simulink model "hw6"  (R2017a)
settings: Solver=VariableStepAuto  StartTime=0.0  StopTime=10.0  RelTol=1e-3
settings Model: Creator=Jessica  LastModifiedBy=Jessica

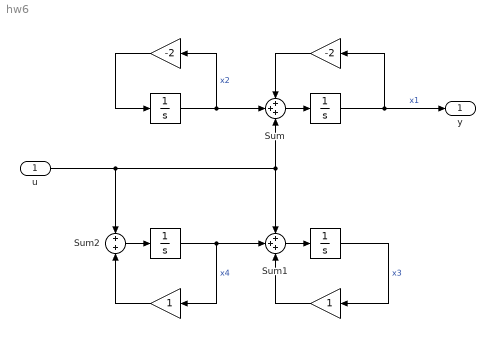
== system hw6 ==
  u : Inport
  " " : Gain  Gain=-2
  "  " : Integrator
  "   " : Integrator
  "    " : Gain  Gain=-2
  "      " : Integrator
  "       " : Gain
  "        " : Gain
  "         " : Integrator
  Sum : Sum  Inputs=+++
  Sum1 : Sum  Inputs=+++
  Sum2 : Sum  Inputs=+|+
  y : Outport
  wires:
  "        "/1 -> Sum2/2
  "         "/1 -> Sum1/2, "        "/1  "x4"
  Sum2/1 -> "         "/1
  "       "/1 -> Sum1/3
  Sum1/1 -> "      "/1
  Sum/1 -> "   "/1
  "    "/1 -> Sum/1
  "  "/1 -> " "/1, Sum/2  "x2"
  " "/1 -> "  "/1
  "   "/1 -> y/1, "    "/1  "x1"
  "      "/1 -> "       "/1  "x3"
  u/1 -> Sum2/1, Sum1/1, Sum/3
